simulink model "Backhoe_Arm"  (R2020a)
settings: Solver=ode23t  StartTime=0.0  StopTime=60  RelTol=1e-3  EnableMultiTasking=on
PostLoadFcn:
  | warning off simscape:compiler:sli:init:SolverNotRecommended
  | 
  | warning off sm:sli:visualization:UnsupportedSimMode
  | warning off sm:sli:setup:compile:LocalSolverNotSupported
  | warning off sm:compiler:state:UnsatisfiedDesiredTarget
  | 
  | warning off xPCTarget:sampleTime:sampleTimeInvariance
  | warning off Simulink:blocks:MatchingFromNotFound
model workspace (MAT data in the model file):
  cylinderGray = [0.6 0.6 0.6]
  darkOrange = [0.8 0.5 0]
  glassBlue = [0.2 0.2 1]
  gray = [0.3 0.3 0.3]
  orange = [0.8 0.65 0]
  pistonGray = [0.4 0.4 0.4]
  rhoGlass = 2500
  rhoRubber = 1500
  rhoSteel = 7800
  tireBlack = [0.1 0.1 0.1]
  wheelGray = [0.6 0.6 0.6]
  yellow = [0.8 0.8 0]
undefined symbols (not defined in the file or in its folder): BH_Param, sigbuilder_block, X, Y, Z
libraries: sm_lib x98, fl_lib x31, Backhoe_Lib x28, nesl_utility x22, sh_lib x9, slrtlib x1
(part 3 of 4)

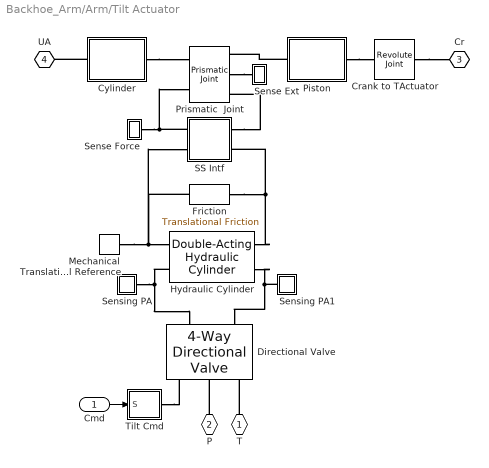
== system Backhoe_Arm/Arm/Tilt Actuator ==
  Cmd : Inport
  Crank to TActuator : sm_lib/Joints/Revolute Joint  JointMode=Normal  SenseConstraintForce=off  SenseConstraintForceX=off  SenseConstraintForceY=off  SenseConstraintForceZ=off  SenseConstraintTorque=off  SenseConstraintTorqueX=off  SenseConstraintTorqueY=off  SenseConstraintTorqueZ=off  SenseTotalForce=off  SenseTotalForceX=off  SenseTotalForceY=off  SenseTotalForceZ=off  SenseTotalTorque=off  SenseTotalTorqueX=off  SenseTotalTorqueY=off  SenseTotalTorqueZ=off  CompositeWrenchDir=FollowerOnBase  CompositeWrenchFrame=BaseFrame  EquilibriumPosition=0  EquilibriumPositionUnits=deg  SpringStiffness=0  SpringStiffnessUnits=N*m/deg  DampingCoefficient=0  DampingCoefficientUnits=N*m/(deg/s)  TorqueActuationMode=NoTorque  MotionActuationMode=ComputedMotion  SensePosition=off  SenseVelocity=off  SenseAcceleration=off  SenseTorqueForce=off  SenseLowerLimitTorqueForce=off  SenseUpperLimitTorqueForce=off  LowerLimitSpecify=off  LowerLimitBound=-90  LowerLimitBoundUnits=deg  LowerLimitStiffness=1e4  LowerLimitStiffnessUnits=N*m/deg  LowerLimitDamping=10  LowerLimitDampingUnits=N*m/(deg/s)  LowerLimitTransitionRegionWidth=0.1  LowerLimitTransitionRegionWidthUnits=deg  UpperLimitSpecify=off  UpperLimitBound=90  UpperLimitBoundUnits=deg  UpperLimitStiffness=1e4  UpperLimitStiffnessUnits=N*m/deg  UpperLimitDamping=10  UpperLimitDampingUnits=N*m/(deg/s)  UpperLimitTransitionRegionWidth=0.1  UpperLimitTransitionRegionWidthUnits=deg  PositionTargetSpecify=off  PositionTargetPriority=High  PositionTargetValue=0  PositionTargetValueUnits=deg  VelocityTargetSpecify=off  VelocityTargetPriority=High  VelocityTargetValue=0  VelocityTargetValueUnits=deg/s
  Cylinder : Subsystem
  Directional Valve : sh_lib/Valves/Directional Valves/4-Way Directional Valve  Tag=Factory Generic  area_spec=1  x_0_P_A=-1e-4 m  x_0_P_B=-1e-4 m  x_0_A_T=-1e-4 m  x_0_B_T=-1e-4 m  mdl_type_identical=1  mdl_type_different=1  opening_max=hydr_valve_max_opening m  area_max=hydr_valve_max_area mm^2  opening_max_P_A=0.005 m  area_max_P_A=0.5e-4 m^2  opening_max_P_B=0.005 m  area_max_P_B=0.5e-4 m^2  opening_max_A_T=0.005 m  area_max_A_T=0.5e-4 m^2  opening_max_B_T=0.005 m  area_max_B_T=0.5e-4 m^2  opening_area_tab="[  -0.002 0 0.005 0.015 ] m"  area_tab="[  1e-12 4e-12 1e-05 1.02e-05 ] m^2"  opening_flow_rate_tab="[  -0.002 0 0.005 0.015 ] m"  pressure_tab="[  -5e+06 -2e+06 2e+06 5e+06 ] Pa"  flow_rate_tab="[  -1e-12 -6e-14 6e+12 1e+11 ; -8e-08 -4e-08 4e+06 8e+06 ; -0.0025 -0.00103 0.001 0.0024 ; -0.00258 -0.001032 0.00106 0.00247 ; ] m^3/s"  opening_area_tab_P_A=[-0.002, 0.0, 0.002, 0.005, 0.015] m  area_tab_P_A=[1.0e-9, 2.0352e-7, 4.0736e-5, 0.00011438, 0.00034356] m^2  opening_flow_rate_tab_P_A=[-0.002, 0.0, 0.002, 0.005, 0.015] m  pressure_tab_P_A=[-10000000.0, -5000000.0, -2000000.0, 2000000.0, 5000000.0, 10000000.0] Pa  flow_rate_tab_P_A=[-1.0e-7, -7.0711e-8, -4.4721e-8, 4.4721e-8, 7.0711e-8, 1.0e-7; -2.0352e-5, -1.4391e-5, -9.1017e-6, 9.1017e-6, 1.4391e-5, 2.0352e-5; -0.0040736, -0.0028805, -0.0018218, 0.0018218, 0.0028805, 0.0040736; -0.011438, -0.0080879, -0.0051152, 0.0051152, 0.0080879, 0.011438; -0.034356, -0.024293, -0.015364, 0.015364, 0.024293, 0.034356] m^3/s  opening_area_tab_P_B=[-0.002, 0.0, 0.002, 0.005, 0.015] m  area_tab_P_B=[1.0e-9, 2.0352e-7, 4.0736e-5, 0.00011438, 0.00034356] m^2  opening_flow_rate_tab_P_B=[-0.002, 0.0, 0.002, 0.005, 0.015] m  pressure_tab_P_B=[-10000000.0, -5000000.0, -2000000.0, 2000000.0, 5000000.0, 10000000.0] Pa  flow_rate_tab_P_B=[-1.0e-7, -7.0711e-8, -4.4721e-8, 4.4721e-8, 7.0711e-8, 1.0e-7; -2.0352e-5, -1.4391e-5, -9.1017e-6, 9.1017e-6, 1.4391e-5, 2.0352e-5; -0.0040736, -0.0028805, -0.0018218, 0.0018218, 0.0028805, 0.0040736; -0.011438, -0.0080879, -0.0051152, 0.0051152, 0.0080879, 0.011438; -0.034356, -0.024293, -0.015364, 0.015364, 0.024293, 0.034356] m^3/s  opening_area_tab_A_T=[-0.002, 0.0, 0.002, 0.005, 0.015] m  area_tab_A_T=[1.0e-9, 2.0352e-7, 4.0736e-5, 0.00011438, 0.00034356] m^2  opening_flow_rate_tab_A_T=[-0.002, 0.0, 0.002, 0.005, 0.015] m  pressure_tab_A_T=[-10000000.0, -5000000.0, -2000000.0, 2000000.0, 5000000.0, 10000000.0] Pa  flow_rate_tab_A_T=[-1.0e-7, -7.0711e-8, -4.4721e-8, 4.4721e-8, 7.0711e-8, 1.0e-7; -2.0352e-5, -1.4391e-5, -9.1017e-6, 9.1017e-6, 1.4391e-5, 2.0352e-5; -0.0040736, -0.0028805, -0.0018218, 0.0018218, 0.0028805, 0.0040736; -0.011438, -0.0080879, -0.0051152, 0.0051152, 0.0080879, 0.011438; -0.034356, -0.024293, -0.015364, 0.015364, 0.024293, 0.034356] m^3/s  opening_area_tab_B_T=[-0.002, 0.0, 0.002, 0.005, 0.015] m  area_tab_B_T=[1.0e-9, 2.0352e-7, 4.0736e-5, 0.00011438, 0.00034356] m^2  opening_flow_rate_tab_B_T=[-0.002, 0.0, 0.002, 0.005, 0.015] m  pressure_tab_B_T=[-10000000.0, -5000000.0, -2000000.0, 2000000.0, 5000000.0, 10000000.0] Pa  flow_rate_tab_B_T=[-1.0e-7, -7.0711e-8, -4.4721e-8, 4.4721e-8, 7.0711e-8, 1.0e-7; -2.0352e-5, -1.4391e-5, -9.1017e-6, 9.1017e-6, 1.4391e-5, 2.0352e-5; -0.0040736, -0.0028805, -0.0018218, 0.0018218, 0.0028805, 0.0040736; -0.011438, -0.0080879, -0.0051152, 0.0051152, 0.0080879, 0.011438; -0.034356, -0.024293, -0.015364, 0.015364, 0.024293, 0.034356] m^3/s  interp_method_identical=1  interp_method_different=1  extrap_method_identical=1  extrap_method_different=1  A_leak=1e-12 m^2  C_d=0.7  lam_spec=2  B_lam=0.999  Re_cr=12
      settings: SourceProductBaseCode=SH  InternalSimscapePortConfiguration="{\"Bottom\":[],\"Left\":[{\"id\":\"A\",\"label\":\"A\",\"type\":\"foundation.hydraulic.hydraulic\"},{\"id\":\"B\",\"label\":\"B\",\"type\":\"foundation.hydraulic.hydraulic\"}],\"Right\":[{\"id\":\"S\",\"label\":\"S\",\"type\":\"input\"},{\"id\":\"P\",\"label\":\"P\",\"type\":\"foundation.hydraulic.hydraulic\"},{\"id\":\"T\",\"label\":\"T\",\"type\":\"foundation.hydraulic.hydraulic\"}],\"Top\":[]}"
  Friction : fl_lib/Mechanical/Translational Elements/Translational Friction  brkwy_frc=friction_breakaway N  brkwy_vel=0.060623 m/s  Col_frc=friction_coulomb N  visc_coef=friction_viscous N/(m/s)  v_specify=off  v_priority=High  v=0 m/s  v_nominal_specify=off  v_nominal_unit=m/s  v_nominal_value=1  f_specify=off  f_priority=High  f=0 N  f_nominal_specify=off  f_nominal_unit=N  f_nominal_value=1
      settings: SourceProductBaseCode=SS  InternalSimscapePortConfiguration="{\"Bottom\":[],\"Left\":[{\"id\":\"R\",\"label\":\"R\",\"type\":\"foundation.mechanical.translational.translational\"}],\"Right\":[{\"id\":\"C\",\"label\":\"C\",\"type\":\"foundation.mechanical.translational.translational\"}],\"Top\":[]}"
  Hydraulic Cylinder : sh_lib/Hydraulic Cylinders/Double-Acting Hydraulic Cylinder  Tag=Factory Generic  area_A=hydr_area m^2  area_B=hydr_area m^2  stroke=hydr_stroke m  init_pos=hydr_x0 m  dead_vol_A=hydr_deadvol m^3  dead_vol_B=hydr_deadvol m^3  init_pressure_A=hydr_PA0 Pa  init_pressure_B=hydr_PB0 Pa  k_sh=1.4  stiff=1e+06 N/m  D=150 N/(m/s)  hardstop_model=3  transition=0.1 mm  or=2
      settings: SourceProductBaseCode=SH  InternalSimscapePortConfiguration="{\"Bottom\":[],\"Left\":[{\"id\":\"C\",\"label\":\"C\",\"type\":\"foundation.mechanical.translational.translational\"},{\"id\":\"A\",\"label\":\"A\",\"type\":\"foundation.hydraulic.hydraulic\"}],\"Right\":[{\"id\":\"R\",\"label\":\"R\",\"type\":\"foundation.mechanical.translational.translational\"},{\"id\":\"B\",\"label\":\"B\",\"type\":\"foundation.hydraulic.hydraulic\"}],\"Top\":[]}"
  Mechanical Translational Reference : fl_lib/Mechanical/Translational Elements/Mechanical Translational Reference  Tag=Factory Generic
  Piston : Subsystem
  Prismatic  Joint : sm_lib/Joints/Prismatic Joint  JointMode=Normal  SenseConstraintForce=off  SenseConstraintForceX=off  SenseConstraintForceY=off  SenseConstraintForceZ=off  SenseConstraintTorque=off  SenseConstraintTorqueX=off  SenseConstraintTorqueY=off  SenseConstraintTorqueZ=off  SenseTotalForce=off  SenseTotalForceX=off  SenseTotalForceY=off  SenseTotalForceZ=off  SenseTotalTorque=off  SenseTotalTorqueX=off  SenseTotalTorqueY=off  SenseTotalTorqueZ=off  CompositeWrenchDir=FollowerOnBase  CompositeWrenchFrame=BaseFrame  EquilibriumPosition=0  EquilibriumPositionUnits=m  SpringStiffness=0  SpringStiffnessUnits=N/m  DampingCoefficient=0  DampingCoefficientUnits=N/(m/s)  TorqueActuationMode=InputTorque  MotionActuationMode=ComputedMotion  SensePosition=on  SenseVelocity=on  SenseAcceleration=off  SenseTorqueForce=off  SenseLowerLimitTorqueForce=off  SenseUpperLimitTorqueForce=off  LowerLimitSpecify=off  LowerLimitBound=-1  LowerLimitBoundUnits=m  LowerLimitStiffness=1e6  LowerLimitStiffnessUnits=N/m  LowerLimitDamping=1e3  LowerLimitDampingUnits=N/(m/s)  LowerLimitTransitionRegionWidth=1e-4  LowerLimitTransitionRegionWidthUnits=m  UpperLimitSpecify=off  UpperLimitBound=1  UpperLimitBoundUnits=m  UpperLimitStiffness=1e6  UpperLimitStiffnessUnits=N/m  UpperLimitDamping=1e3  UpperLimitDampingUnits=N/(m/s)  UpperLimitTransitionRegionWidth=1e-4  UpperLimitTransitionRegionWidthUnits=m  PositionTargetSpecify=off  PositionTargetPriority=Low  PositionTargetValue=0  PositionTargetValueUnits=m  VelocityTargetSpecify=off  VelocityTargetPriority=High  VelocityTargetValue=0  VelocityTargetValueUnits=m/s
  SS Intf : Subsystem
  Sense Ext : Subsystem
      mask Display: disp('S')
  Sense Force : Subsystem
      mask Display: disp('S')
  Sensing PA : Subsystem
      mask Display: disp('S')
  Sensing PA1 : Subsystem
      mask Display: disp('S')
  Tilt Cmd : Subsystem
  T : PMIOPort  Side=Left
  P : PMIOPort  Port=2  Side=Left
  Cr : PMIOPort  Port=3  Side=Right
  UA : PMIOPort  Port=4  Side=Right
  wires:
  Cmd/1 -> Tilt Cmd/1(S)
  connections:
  Crank to TActuator/RConn1 -- Cr/RConn1
  SS Intf/RConn1 -- Sense Force/RConn1 -- Prismatic  Joint/LConn2
  SS Intf/LConn1 -- Prismatic  Joint/RConn3
  Piston/LConn1 -- Prismatic  Joint/RConn1
  Cylinder/LConn1 -- Prismatic  Joint/LConn1
  Hydraulic Cylinder/RConn1 -- Friction/LConn1 -- SS Intf/LConn2
  Sensing PA/LConn1 -- Hydraulic Cylinder/LConn2 -- Directional Valve/LConn1
  Mechanical Translational Reference/LConn1 -- Friction/RConn1 -- SS Intf/RConn2 -- Hydraulic Cylinder/LConn1
  Hydraulic Cylinder/RConn2 -- Sensing PA1/LConn1 -- Directional Valve/LConn2
  Cylinder/RConn1 -- UA/RConn1
  P/RConn1 -- Directional Valve/RConn2
  T/RConn1 -- Directional Valve/RConn3
  Tilt Cmd/RConn1 -- Directional Valve/RConn1
  Prismatic  Joint/RConn2 -- Sense Ext/LConn1
  Piston/RConn1 -- Crank to TActuator/LConn1

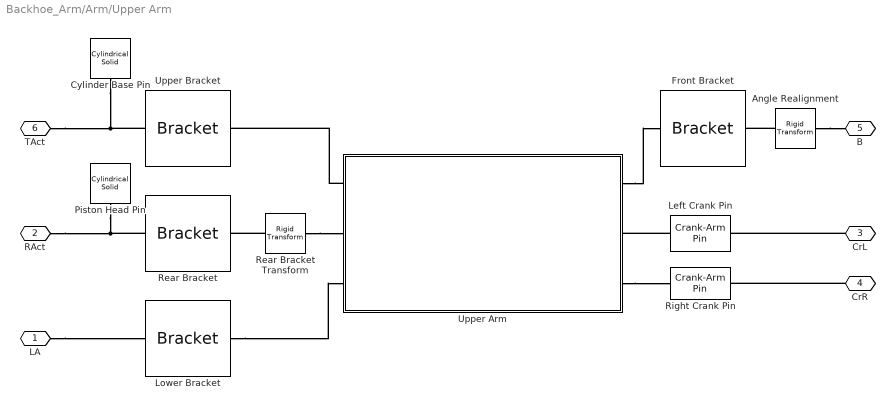
== system Backhoe_Arm/Arm/Upper Arm ==
  Angle Realignment : sm_lib/Frames and Transforms/Rigid Transform  TranslationMethod=None  TranslationStandardOffset=0  TranslationLengthUnit=m  TranslationStandardAxis=+Z  TranslationCartesianOffset=[0 0 0]  TranslationROffset=0  TranslationROffsetUnits=m  TranslationZOffset=0  TranslationZOffsetUnits=m  TranslationThetaOffset=0  TranslationThetaOffsetUnits=deg  RotationMethod=AlignedAxes  RotationAngleUnits=deg  RotationStandardAxis=-Z  RotationAngle=90  RotationArbitraryAxis=[0 0 1]  FollAlignAxisA=+X  BaseAlignAxisA=-Y  FollAlignAxisB=+Z  BaseAlignAxisB=+Z  RotationSequenceAxes=FollowerAxes  RotationSequence=XYX  RotationSequenceAngles=[0 0 0]  RotationSequenceAnglesUnits=deg  RotationMatrix=[1 0 0; 0 1 0; 0 0 1]
  Cylinder Base Pin : sm_lib/Body Elements/Cylindrical Solid  GraphicAmbientColor=[0.15 0.15 0.15 1.0]  BasedOnType=Density  CenterOfMass=[0 0 0]  CenterOfMassUnits=m  GraphicDiffuseColor=gray  CylinderLength=0.8  CylinderLengthUnits=m  CylinderRadius=0.075  CylinderRadiusUnits=m  Density=rhoSteel  DensityUnits=kg/(m^3)  DoExposeReferenceFrame=on  GraphicEmissiveColor=[0.0 0.0 0.0 1.0]  ExportEntireGeometry=off  SerializedFrames=<Frames/>  MarkerShape=Sphere  MarkerSize=10  GraphicType=FromGeometry  InertiaType=CalculateFromGeometry  Mass=1  MassUnits=kg  MomentsOfInertia=[1 1 1]  MomentsOfInertiaUnits=kg*m^2  GraphicOpacity=1.0  ProductsOfInertia=[0 0 0]  ProductsOfInertiaUnits=kg*m^2  GraphicShininess=75  GraphicSpecularColor=[0.5 0.5 0.5 1.0]  GraphicVisPropType=SimpleVisualProperties
  Front Bracket : Backhoe_Lib/Bracket  Hbracket=0.65  Wbracket=0.5  Tbracket=0.15  Dbracket=0.625  Hhole=0.4  Rhole=0.075  circlePoints=25  bracketColor=orange  rho=rhoSteel
  Left Crank Pin : Backhoe_Lib/Crank-Arm Pin  R=0.075  L=0.25  T=0.2  color=gray  rho=rhoSteel
  Lower Bracket : Backhoe_Lib/Bracket  Hbracket=0.75  Wbracket=0.75  Tbracket=0.15  Dbracket=0.75  Hhole=0.5  Rhole=0.075  circlePoints=25  bracketColor=orange  rho=rhoSteel
  Piston Head Pin : sm_lib/Body Elements/Cylindrical Solid  GraphicAmbientColor=[0.15 0.15 0.15 1.0]  BasedOnType=Density  CenterOfMass=[0 0 0]  CenterOfMassUnits=m  GraphicDiffuseColor=gray  CylinderLength=0.8  CylinderLengthUnits=m  CylinderRadius=0.075  CylinderRadiusUnits=m  Density=rhoSteel  DensityUnits=kg/(m^3)  DoExposeReferenceFrame=on  GraphicEmissiveColor=[0.0 0.0 0.0 1.0]  ExportEntireGeometry=off  SerializedFrames=<Frames/>  MarkerShape=Sphere  MarkerSize=10  GraphicType=FromGeometry  InertiaType=CalculateFromGeometry  Mass=1  MassUnits=kg  MomentsOfInertia=[1 1 1]  MomentsOfInertiaUnits=kg*m^2  GraphicOpacity=1.0  ProductsOfInertia=[0 0 0]  ProductsOfInertiaUnits=kg*m^2  GraphicShininess=75  GraphicSpecularColor=[0.5 0.5 0.5 1.0]  GraphicVisPropType=SimpleVisualProperties
  Rear Bracket : Backhoe_Lib/Bracket  Hbracket=0.75  Wbracket=0.75  Tbracket=0.15  Dbracket=0.75  Hhole=0.5  Rhole=0.075  circlePoints=25  bracketColor=orange  rho=rhoSteel
  Rear Bracket Transform : sm_lib/Frames and Transforms/Rigid Transform  TranslationMethod=None  TranslationStandardOffset=0.5  TranslationLengthUnit=m  TranslationStandardAxis=+Z  TranslationCartesianOffset=[ 0 0 0]  TranslationROffset=0  TranslationROffsetUnits=m  TranslationZOffset=0  TranslationZOffsetUnits=m  TranslationThetaOffset=0  TranslationThetaOffsetUnits=deg  RotationMethod=AlignedAxes  RotationAngleUnits=deg  RotationStandardAxis=+X  RotationAngle=90  RotationArbitraryAxis=[0 0 1]  FollAlignAxisA=+Z  BaseAlignAxisA=+Z  FollAlignAxisB=+Y  BaseAlignAxisB=-Y  RotationSequenceAxes=FollowerAxes  RotationSequence=XYX  RotationSequenceAngles=[0 0 0]  RotationSequenceAnglesUnits=deg  RotationMatrix=[1 0 0; 0 1 0; 0 0 1]
  Right Crank Pin : Backhoe_Lib/Crank-Arm Pin  R=0.075  L=0.25  T=0.2  color=gray  rho=rhoSteel
  Upper Arm : Subsystem  mask(Upper Arm){Lbar=6, Wbar=0.8, Tbar=0.85, L1=1.5, L2=1.5, L3=2.5, barFillet=0.1, numPoints=15, Tcrank=0.2, armColor=yellow, rho=rhoSteel}
      mask prompts: Lbar "Lbar [m]"; Wbar "Wbar [m]"; Tbar "Tbar [m]"; L1 "L1 [m]"; L2 "L2 [m]"; L3 "L3 [m]"; barFillet "Bar Fillet Radius [m]"; numPoints "Fillet Point Resolution"; Tcrank "Crank Arm Thickness [m]"; armColor "Arm Color"; rho "Density [kg/m^3]"
      mask help:
      | Consists of the backhoe upper arm and four attachment brackets -- front, rear, upper and lower.
      |
      | Attachment points are:
      | B: Bucket attachment.
      | CL: Crank arm attachment (Left).
      | CR: Crank arm attachment (Right).
      | BC: Bucket hydraulic actuator (Cylinder base).
      | LA: Lower Arm attachment.
      | UH: Upper arm hydraulic actuator (piston Head).
      | All attachment points are configured for Revolute joints.
      |
      | The lengths L1, L2 and L3 correspond to lengths measured from the center of the bar, as follows:
      | L1: Upper Bracket
      | L2: Lower Bracket
      | L3: Crank Attachment Points
      | The front and rear brackets are automatically placed at the center of the end faces of the upper arm bar.
      |
      | Click on Help to view a schematic of the upper arm, its configurable dimension parameters and attachment points (in red).
      mask init: same as Backhoe_Arm/Arm/Lower Arm /Lower Arm
      mask Help: web('Backhoe_Upperarm.html');
      mask DialogControl ParameterTabVar0 Prompt: General
      mask DialogControl ParameterTabVar01 Prompt: Material Properties
      mask Display:
      | image('Backhoe_Upperbar_IMAGE.png');
      | port_label('lconn',1,'CB');
      | port_label('lconn',2,'PH');
      | port_label('lconn',3,'LA');
      | port_label('rconn',1,'B');
      | port_label('rconn',2,'CL');
      | port_label('rconn',3,'CR');
  Upper Bracket : Backhoe_Lib/Bracket  Hbracket=0.75  Wbracket=0.75  Tbracket=0.15  Dbracket=0.75  Hhole=0.5  Rhole=0.075  circlePoints=25  bracketColor=orange  rho=rhoSteel
  LA : PMIOPort  Side=Left
  RAct : PMIOPort  Port=2  Side=Left
  CrL : PMIOPort  Port=3  Side=Right
  CrR : PMIOPort  Port=4  Side=Right
  B : PMIOPort  Port=5  Side=Right
  TAct : PMIOPort  Port=6  Side=Right
  connections:
  Cylinder Base Pin/RConn1 -- Upper Bracket/RConn1 -- TAct/RConn1
  Piston Head Pin/RConn1 -- RAct/RConn1 -- Rear Bracket/RConn1
  Angle Realignment/LConn1 -- Front Bracket/RConn1
  LA/RConn1 -- Lower Bracket/RConn1
  CrL/RConn1 -- Left Crank Pin/LConn1
  CrR/RConn1 -- Right Crank Pin/LConn1
  Rear Bracket Transform/RConn1 -- Rear Bracket/LConn1
  Upper Arm/LConn1 -- Upper Bracket/LConn1
  Upper Arm/RConn1 -- Front Bracket/LConn1
  Upper Arm/RConn3 -- Right Crank Pin/RConn1
  Lower Bracket/LConn1 -- Upper Arm/LConn3
  Rear Bracket Transform/LConn1 -- Upper Arm/LConn2
  Left Crank Pin/RConn1 -- Upper Arm/RConn2
  Angle Realignment/RConn1 -- B/RConn1

== system Backhoe_Arm/Arm/Bucket Assembly/Bucket ==
  Arm Revolute Rotation : sm_lib/Frames and Transforms/Rigid Transform  TranslationMethod=None  TranslationStandardOffset=0  TranslationLengthUnit=m  TranslationStandardAxis=+X  TranslationCartesianOffset=[0 0 0]  TranslationROffset=0  TranslationROffsetUnits=m  TranslationZOffset=0  TranslationZOffsetUnits=m  TranslationThetaOffset=0  TranslationThetaOffsetUnits=deg  RotationMethod=AlignedAxes  RotationAngleUnits=deg  RotationStandardAxis=-Y  RotationAngle=180  RotationArbitraryAxis=[0 0 1]  FollAlignAxisA=+Y  BaseAlignAxisA=+Y  FollAlignAxisB=+X  BaseAlignAxisB=-X  RotationSequenceAxes=FollowerAxes  RotationSequence=XYX  RotationSequenceAngles=[0 0 0]  RotationSequenceAnglesUnits=deg  RotationMatrix=[1 0 0; 0 1 0; 0 0 1]
  Attachment Frame : Subsystem
      mask Display:
      | image('Backhoe_Attach_IMAGE.png');
      | port_label('lconn',1,'B');
      | port_label('rconn',1,'CA');
      | port_label('rconn',2,'UA');
  Bucket : Subsystem
      mask Display:
      | image('Backhoe_Bucketcase_IMAGE.png');
      | port_label('rconn',1,'AF');
  Crank Revolute Rotation : sm_lib/Frames and Transforms/Rigid Transform  TranslationMethod=None  TranslationStandardOffset=0  TranslationLengthUnit=m  TranslationStandardAxis=+X  TranslationCartesianOffset=[0 0 0]  TranslationROffset=0  TranslationROffsetUnits=m  TranslationZOffset=0  TranslationZOffsetUnits=m  TranslationThetaOffset=0  TranslationThetaOffsetUnits=deg  RotationMethod=AlignedAxes  RotationAngleUnits=deg  RotationStandardAxis=-Y  RotationAngle=180  RotationArbitraryAxis=[0 0 1]  FollAlignAxisA=+Y  BaseAlignAxisA=+Y  FollAlignAxisB=+X  BaseAlignAxisB=-X  RotationSequenceAxes=FollowerAxes  RotationSequence=XYX  RotationSequenceAngles=[0 0 0]  RotationSequenceAnglesUnits=deg  RotationMatrix=[1 0 0; 0 1 0; 0 0 1]
  Crank Arm : PMIOPort  Side=Right
  Upper Arm : PMIOPort  Port=2  Side=Right
  connections:
  Bucket/RConn1 -- Attachment Frame/LConn1
  Crank Revolute Rotation/LConn1 -- Attachment Frame/RConn1
  Arm Revolute Rotation/LConn1 -- Attachment Frame/RConn2
  Upper Arm/RConn1 -- Arm Revolute Rotation/RConn1
  Crank Arm/RConn1 -- Crank Revolute Rotation/RConn1

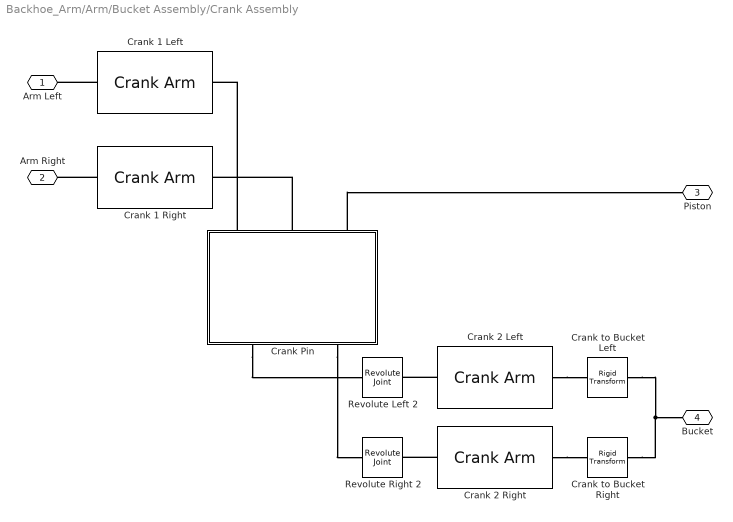
== system Backhoe_Arm/Arm/Bucket Assembly/Crank Assembly ==
  Crank 1 Left : Backhoe_Lib/Crank Arm  L=LC1  W=WC1  T=TC1  D=DH1  R=Rpin  Nc=25  color=color1  rho=rho1
  Crank 1 Right : Backhoe_Lib/Crank Arm  L=LC1  W=WC1  T=TC1  D=DH1  R=Rpin  Nc=25  color=color1  rho=rho1
  Crank 2 Left : Backhoe_Lib/Crank Arm  L=LC2  W=WC2  T=TC2  D=DH2  R=Rpin  Nc=25  color=color2  rho=rho2
  Crank 2 Right : Backhoe_Lib/Crank Arm  L=LC2  W=WC2  T=TC2  D=DH2  R=Rpin  Nc=25  color=color2  rho=rho2
  Crank Pin : Subsystem
      mask Display:
      | image(repmat(imread('Backhoe_Crankpin_IMAGE.png'),[1 1 3]));
      | port_label('lconn',1,'C1L');
      | port_label('lconn',2,'C2L');
      | port_label('lconn',3,'PA');
      | port_label('rconn',1,'C2L');
      | port_label('rconn',2,'C2R');
  Crank to Bucket Right : sm_lib/Frames and Transforms/Rigid Transform  TranslationMethod=StandardAxis  TranslationStandardOffset=(DC2 - TC2)/2  TranslationLengthUnit=m  TranslationStandardAxis=+Z  TranslationCartesianOffset=[0 0 0]  TranslationROffset=0  TranslationROffsetUnits=m  TranslationZOffset=0  TranslationZOffsetUnits=m  TranslationThetaOffset=0  TranslationThetaOffsetUnits=deg  RotationMethod=None  RotationAngleUnits=deg  RotationStandardAxis=+Z  RotationAngle=0  RotationArbitraryAxis=[0 0 1]  FollAlignAxisA=+X  BaseAlignAxisA=+Y  FollAlignAxisB=+Y  BaseAlignAxisB=+Z  RotationSequenceAxes=FollowerAxes  RotationSequence=XYX  RotationSequenceAngles=[0 0 0]  RotationSequenceAnglesUnits=deg  RotationMatrix=[1 0 0; 0 1 0; 0 0 1]
  Crank to Bucket Left : sm_lib/Frames and Transforms/Rigid Transform  TranslationMethod=StandardAxis  TranslationStandardOffset=(DC2 - TC2)/2  TranslationLengthUnit=m  TranslationStandardAxis=-Z  TranslationCartesianOffset=[0 0 0]  TranslationROffset=0  TranslationROffsetUnits=m  TranslationZOffset=0  TranslationZOffsetUnits=m  TranslationThetaOffset=0  TranslationThetaOffsetUnits=deg  RotationMethod=None  RotationAngleUnits=deg  RotationStandardAxis=+Z  RotationAngle=0  RotationArbitraryAxis=[0 0 1]  FollAlignAxisA=+X  BaseAlignAxisA=+Y  FollAlignAxisB=+Y  BaseAlignAxisB=+Z  RotationSequenceAxes=FollowerAxes  RotationSequence=XYX  RotationSequenceAngles=[0 0 0]  RotationSequenceAnglesUnits=deg  RotationMatrix=[1 0 0; 0 1 0; 0 0 1]
  Revolute Left 2 : sm_lib/Joints/Revolute Joint  JointMode=Normal  SenseConstraintForce=off  SenseConstraintForceX=off  SenseConstraintForceY=off  SenseConstraintForceZ=off  SenseConstraintTorque=off  SenseConstraintTorqueX=off  SenseConstraintTorqueY=off  SenseConstraintTorqueZ=off  SenseTotalForce=off  SenseTotalForceX=off  SenseTotalForceY=off  SenseTotalForceZ=off  SenseTotalTorque=off  SenseTotalTorqueX=off  SenseTotalTorqueY=off  SenseTotalTorqueZ=off  CompositeWrenchDir=FollowerOnBase  CompositeWrenchFrame=BaseFrame  EquilibriumPosition=0  EquilibriumPositionUnits=deg  SpringStiffness=0  SpringStiffnessUnits=N*m/deg  DampingCoefficient=0  DampingCoefficientUnits=N*m/(deg/s)  TorqueActuationMode=NoTorque  MotionActuationMode=ComputedMotion  SensePosition=off  SenseVelocity=off  SenseAcceleration=off  SenseTorqueForce=off  SenseLowerLimitTorqueForce=off  SenseUpperLimitTorqueForce=off  LowerLimitSpecify=off  LowerLimitBound=-90  LowerLimitBoundUnits=deg  LowerLimitStiffness=1e4  LowerLimitStiffnessUnits=N*m/deg  LowerLimitDamping=10  LowerLimitDampingUnits=N*m/(deg/s)  LowerLimitTransitionRegionWidth=0.1  LowerLimitTransitionRegionWidthUnits=deg  UpperLimitSpecify=off  UpperLimitBound=90  UpperLimitBoundUnits=deg  UpperLimitStiffness=1e4  UpperLimitStiffnessUnits=N*m/deg  UpperLimitDamping=10  UpperLimitDampingUnits=N*m/(deg/s)  UpperLimitTransitionRegionWidth=0.1  UpperLimitTransitionRegionWidthUnits=deg  PositionTargetSpecify=off  PositionTargetPriority=Low  PositionTargetValue=-45  PositionTargetValueUnits=deg  VelocityTargetSpecify=off  VelocityTargetPriority=High  VelocityTargetValue=0  VelocityTargetValueUnits=deg/s
  Revolute Right 2 : sm_lib/Joints/Revolute Joint  JointMode=Normal  SenseConstraintForce=off  SenseConstraintForceX=off  SenseConstraintForceY=off  SenseConstraintForceZ=off  SenseConstraintTorque=off  SenseConstraintTorqueX=off  SenseConstraintTorqueY=off  SenseConstraintTorqueZ=off  SenseTotalForce=off  SenseTotalForceX=off  SenseTotalForceY=off  SenseTotalForceZ=off  SenseTotalTorque=off  SenseTotalTorqueX=off  SenseTotalTorqueY=off  SenseTotalTorqueZ=off  CompositeWrenchDir=FollowerOnBase  CompositeWrenchFrame=BaseFrame  EquilibriumPosition=0  EquilibriumPositionUnits=deg  SpringStiffness=0  SpringStiffnessUnits=N*m/deg  DampingCoefficient=0  DampingCoefficientUnits=N*m/(deg/s)  TorqueActuationMode=NoTorque  MotionActuationMode=ComputedMotion  SensePosition=off  SenseVelocity=off  SenseAcceleration=off  SenseTorqueForce=off  SenseLowerLimitTorqueForce=off  SenseUpperLimitTorqueForce=off  LowerLimitSpecify=off  LowerLimitBound=-90  LowerLimitBoundUnits=deg  LowerLimitStiffness=1e4  LowerLimitStiffnessUnits=N*m/deg  LowerLimitDamping=10  LowerLimitDampingUnits=N*m/(deg/s)  LowerLimitTransitionRegionWidth=0.1  LowerLimitTransitionRegionWidthUnits=deg  UpperLimitSpecify=off  UpperLimitBound=90  UpperLimitBoundUnits=deg  UpperLimitStiffness=1e4  UpperLimitStiffnessUnits=N*m/deg  UpperLimitDamping=10  UpperLimitDampingUnits=N*m/(deg/s)  UpperLimitTransitionRegionWidth=0.1  UpperLimitTransitionRegionWidthUnits=deg  PositionTargetSpecify=off  PositionTargetPriority=High  PositionTargetValue=0  PositionTargetValueUnits=deg  VelocityTargetSpecify=off  VelocityTargetPriority=High  VelocityTargetValue=0  VelocityTargetValueUnits=deg/s
  Arm Left : PMIOPort  Side=Left
  Arm Right : PMIOPort  Port=2  Side=Left
  Piston : PMIOPort  Port=3  Side=Right
  Bucket : PMIOPort  Port=4  Side=Right
  connections:
  Crank Pin/RConn1 -- Revolute Left 2/LConn1
  Crank Pin/RConn2 -- Revolute Right 2/LConn1
  Crank 2 Left/LConn1 -- Revolute Left 2/RConn1
  Crank to Bucket Right/RConn1 -- Crank to Bucket Left/RConn1 -- Bucket/RConn1
  Crank Pin/LConn3 -- Piston/RConn1
  Crank 1 Left/RConn1 -- Arm Left/RConn1
  Crank 1 Right/RConn1 -- Arm Right/RConn1
  Crank Pin/LConn1 -- Crank 1 Left/LConn1
  Crank Pin/LConn2 -- Crank 1 Right/LConn1
  Crank 2 Right/LConn1 -- Revolute Right 2/RConn1
  Crank 2 Right/RConn1 -- Crank to Bucket Right/LConn1
  Crank 2 Left/RConn1 -- Crank to Bucket Left/LConn1

== system Backhoe_Arm/Arm/Lift Actuator/Cylinder ==
  Base to Cylinder Transform : sm_lib/Frames and Transforms/Rigid Transform  TranslationMethod=StandardAxis  TranslationStandardOffset=(Lcyl/2)  TranslationLengthUnit=m  TranslationStandardAxis=-Z  TranslationCartesianOffset=[0 0 0]  TranslationROffset=0  TranslationROffsetUnits=m  TranslationZOffset=0  TranslationZOffsetUnits=m  TranslationThetaOffset=0  TranslationThetaOffsetUnits=deg  RotationMethod=AlignedAxes  RotationAngleUnits=deg  RotationStandardAxis=+X  RotationAngle=90  RotationArbitraryAxis=[0 0 1]  FollAlignAxisA=+X  BaseAlignAxisA=+X  FollAlignAxisB=+Z  BaseAlignAxisB=-Z  RotationSequenceAxes=FollowerAxes  RotationSequence=XYX  RotationSequenceAngles=[0 0 0]  RotationSequenceAnglesUnits=deg  RotationMatrix=[1 0 0; 0 1 0; 0 0 1]
  Cylinder : sm_lib/Body Elements/Extruded Solid  GraphicAmbientColor=[0.15 0.15 0.15 1.0]  BasedOnType=Density  CenterOfMass=[0 0 0]  CenterOfMassUnits=m  GraphicDiffuseColor=cylColor  ExportConvexHullGeometry=off  ExtrusionCrossSection=cylSection  ExtrusionCrossSectionUnits=m  Density=rhoCyl  DensityUnits=kg/(m^3)  DoExposeReferenceFrame=on  GraphicEmissiveColor=[0.0 0.0 0.0 1.0]  ExportEntireGeometry=off  ExtrusionLength=Lcyl  ExtrusionLengthUnits=m  ExtrusionType=General  SerializedFrames=<Frames/>  MarkerShape=Sphere  MarkerSize=10  GraphicType=FromGeometry  InertiaType=CalculateFromGeometry  Mass=1  MassUnits=kg  MomentsOfInertia=[1 1 1]  MomentsOfInertiaUnits=kg*m^2  PolygonNumSides=3  GraphicOpacity=1  PolygonOuterRadius=1  PolygonOuterRadiusUnits=m  ProductsOfInertia=[0 0 0]  ProductsOfInertiaUnits=kg*m^2  GraphicShininess=75  GraphicSpecularColor=[0.5 0.5 0.5 1.0]  GraphicVisPropType=SimpleVisualProperties
  Single Bracket : Backhoe_Lib/Single Bracket  Hbracket=Lbase  Wbracket=Wbase  Tbracket=Wbase  Hhole=Lbase-(Wbase/2)  Rhole=Rbp  Nc=25  bracketColor=connColor  rho=rhoConn
  F : PMIOPort  Side=Right
  B : PMIOPort  Port=2  Side=Left
  connections:
  Single Bracket/RConn1 -- F/RConn1
  Single Bracket/LConn1 -- Base to Cylinder Transform/RConn1
  Cylinder/RConn1 -- Base to Cylinder Transform/LConn1 -- B/RConn1

== system Backhoe_Arm/Arm/Lift Actuator/Lift ==
  S : Inport
  Lift Cmd : Selector  InputPortWidth=3  IndexOptions=Index vector (dialog)  Indices=3  OutputSizes=1
  Simulink-PS Converter : nesl_utility/Simulink-PS Converter  PhysicalDomain=network_engine_domain  SubClassName=ps_input  LeftPortType=input  RightPortType=output  PseudoPeriodic=off  Frequencies=[]  NoiseDistribution=none  NoiseParameters=[]  Unit=1  AffineConversion=off  FilteringAndDerivatives=zero  SimscapeFilterOrder=1  InputFilterTimeConstant=0.005  UdotUserProvided=0
  PS : PMIOPort  Side=Right
  wires:
  Lift Cmd/1 -> Simulink-PS Converter/1
  S/1 -> Lift Cmd/1
  connections:
  PS/RConn1 -- Simulink-PS Converter/RConn1

== system Backhoe_Arm/Arm/Lift Actuator/Piston ==
  Piston : sm_lib/Body Elements/Cylindrical Solid  GraphicAmbientColor=[0.15 0.15 0.15 1.0]  BasedOnType=Density  CenterOfMass=[0 0 0]  CenterOfMassUnits=m  GraphicDiffuseColor=pistColor  CylinderLength=Lpist  CylinderLengthUnits=m  CylinderRadius=Rpist  CylinderRadiusUnits=m  Density=rhoPist  DensityUnits=kg/(m^3)  DoExposeReferenceFrame=on  GraphicEmissiveColor=[0.0 0.0 0.0 1.0]  ExportEntireGeometry=off  SerializedFrames=<Frames/>  MarkerShape=Sphere  MarkerSize=10  GraphicType=FromGeometry  InertiaType=CalculateFromGeometry  Mass=1  MassUnits=kg  MomentsOfInertia=[1 1 1]  MomentsOfInertiaUnits=kg*m^2  GraphicOpacity=1.0  ProductsOfInertia=[0 0 0]  ProductsOfInertiaUnits=kg*m^2  GraphicShininess=75  GraphicSpecularColor=[0.5 0.5 0.5 1.0]  GraphicVisPropType=SimpleVisualProperties
  Piston to Head Transform : sm_lib/Frames and Transforms/Rigid Transform  TranslationMethod=StandardAxis  TranslationStandardOffset=Lpist/2  TranslationLengthUnit=m  TranslationStandardAxis=+Z  TranslationCartesianOffset=[0 0 0]  TranslationROffset=0  TranslationROffsetUnits=m  TranslationZOffset=0  TranslationZOffsetUnits=m  TranslationThetaOffset=0  TranslationThetaOffsetUnits=deg  RotationMethod=AlignedAxes  RotationAngleUnits=deg  RotationStandardAxis=-X  RotationAngle=90  RotationArbitraryAxis=[0 0 1]  FollAlignAxisA=+Y  BaseAlignAxisA=-Y  FollAlignAxisB=+Z  BaseAlignAxisB=+Z  RotationSequenceAxes=FollowerAxes  RotationSequence=XYX  RotationSequenceAngles=[0 0 0]  RotationSequenceAnglesUnits=deg  RotationMatrix=[1 0 0; 0 1 0; 0 0 1]
  Single Bracket : Backhoe_Lib/Single Bracket  Hbracket=Lbase  Wbracket=Wbase  Tbracket=Whead  Hhole=Lhead-(Whead/2)  Rhole=Rhp  Nc=25  bracketColor=connColor  rho=rhoConn
  B : PMIOPort  Side=Left
  F : PMIOPort  Port=2  Side=Right
  connections:
  Single Bracket/RConn1 -- F/RConn1
  Piston to Head Transform/RConn1 -- Single Bracket/LConn1
  B/RConn1 -- Piston to Head Transform/LConn1 -- Piston/RConn1

== system Backhoe_Arm/Arm/Lift Actuator/SS Intf ==
  Ideal Force Sensor : fl_lib/Mechanical/Mechanical Sensors/Ideal Force Sensor
  Ideal Translational Velocity Source : fl_lib/Mechanical/Mechanical Sources/Ideal Translational Velocity Source
  F : PMIOPort  Side=Right
  V : PMIOPort  Port=2  Side=Left
  R : PMIOPort  Port=3  Side=Left
  C : PMIOPort  Port=4  Side=Right
  connections:
  Ideal Force Sensor/RConn2 -- F/RConn1
  Ideal Force Sensor/LConn1 -- R/RConn1
  C/RConn1 -- Ideal Translational Velocity Source/RConn2
  V/RConn1 -- Ideal Translational Velocity Source/RConn1
  Ideal Force Sensor/RConn1 -- Ideal Translational Velocity Source/LConn1

== system Backhoe_Arm/Arm/Lift Actuator/Sense Ext ==
  PS-Simulink Converter : nesl_utility/PS-Simulink Converter  PhysicalDomain=network_engine_domain  SubClassName=ps_output  LeftPortType=input  RightPortType=output  PseudoPeriodic=off  Frequencies=[]  Unit=1  AffineConversion=off
  Conn1 : PMIOPort  Side=Left
  tag scope: Lift_Ext=global
  wires:
  PS-Simulink Converter/1 -> [Lift_Ext]
  connections:
  Conn1/RConn1 -- PS-Simulink Converter/LConn1

== system Backhoe_Arm/Arm/Lift Actuator/Sense Force ==
  PS-Simulink Converter : nesl_utility/PS-Simulink Converter  PhysicalDomain=network_engine_domain  SubClassName=ps_output  LeftPortType=input  RightPortType=output  PseudoPeriodic=off  Frequencies=[]  Unit=1  AffineConversion=off
  S : PMIOPort  Side=Right
  tag scope: Lift_Force=global
  wires:
  PS-Simulink Converter/1 -> [Lift_Force]
  connections:
  PS-Simulink Converter/LConn1 -- S/RConn1

== system Backhoe_Arm/Arm/Lift Actuator/Sensing PA ==
  Hydraulic Pressure Sensor : fl_lib/Hydraulic/Hydraulic Sensors/Hydraulic Pressure Sensor
  Hydraulic Reference : fl_lib/Hydraulic/Hydraulic Elements/Hydraulic Reference
  PS-Simulink Converter1 : nesl_utility/PS-Simulink Converter  PhysicalDomain=network_engine_domain  SubClassName=ps_output  LeftPortType=input  RightPortType=output  PseudoPeriodic=off  Frequencies=[]  Unit=Pa  AffineConversion=off
  A : PMIOPort  Side=Left
  tag scope: Lift_PA=global
  wires:
  PS-Simulink Converter1/1 -> [Lift_PA]
  connections:
  Hydraulic Pressure Sensor/LConn1 -- A/RConn1
  Hydraulic Reference/LConn1 -- Hydraulic Pressure Sensor/RConn1
  PS-Simulink Converter1/LConn1 -- Hydraulic Pressure Sensor/RConn2

== system Backhoe_Arm/Arm/Lift Actuator/Sensing PA1 ==
  Hydraulic Pressure Sensor : fl_lib/Hydraulic/Hydraulic Sensors/Hydraulic Pressure Sensor
  Hydraulic Reference1 : fl_lib/Hydraulic/Hydraulic Elements/Hydraulic Reference
  PS-Simulink Converter1 : nesl_utility/PS-Simulink Converter  PhysicalDomain=network_engine_domain  SubClassName=ps_output  LeftPortType=input  RightPortType=output  PseudoPeriodic=off  Frequencies=[]  Unit=Pa  AffineConversion=off
  A : PMIOPort  Side=Left
  tag scope: Lift_PB=global
  wires:
  PS-Simulink Converter1/1 -> [Lift_PB]
  connections:
  PS-Simulink Converter1/LConn1 -- Hydraulic Pressure Sensor/RConn2
  Hydraulic Reference1/LConn1 -- Hydraulic Pressure Sensor/RConn1
  Hydraulic Pressure Sensor/LConn1 -- A/RConn1

== system Backhoe_Arm/Arm/Lower Arm /Lower Arm ==
  Bar : sm_lib/Body Elements/Extruded Solid  GraphicAmbientColor=[0.15 0.15 0.15 1.0]  BasedOnType=Density  CenterOfMass=[0 0 0]  CenterOfMassUnits=m  GraphicDiffuseColor=armColor  ExportConvexHullGeometry=off  ExtrusionCrossSection=barSection  ExtrusionCrossSectionUnits=m  Density=rho  DensityUnits=kg/(m^3)  DoExposeReferenceFrame=on  GraphicEmissiveColor=[0.0 0.0 0.0 1.0]  ExportEntireGeometry=off  ExtrusionLength=Lbar  ExtrusionLengthUnits=m  ExtrusionType=General  SerializedFrames=<Frames/>  MarkerShape=Sphere  MarkerSize=10  GraphicType=FromGeometry  InertiaType=CalculateFromGeometry  Mass=1  MassUnits=kg  MomentsOfInertia=[1 1 1]  MomentsOfInertiaUnits=kg*m^2  PolygonNumSides=3  GraphicOpacity=1.0  PolygonOuterRadius=1  PolygonOuterRadiusUnits=m  ProductsOfInertia=[0 0 0]  ProductsOfInertiaUnits=kg*m^2  GraphicShininess=75  GraphicSpecularColor=[0.5 0.5 0.5 1.0]  GraphicVisPropType=SimpleVisualProperties
  Front Bracket Transform : sm_lib/Frames and Transforms/Rigid Transform  TranslationMethod=StandardAxis  TranslationStandardOffset=Lbar/2  TranslationLengthUnit=m  TranslationStandardAxis=+Z  TranslationCartesianOffset=[0 0 0]  TranslationROffset=0  TranslationROffsetUnits=m  TranslationZOffset=0  TranslationZOffsetUnits=m  TranslationThetaOffset=0  TranslationThetaOffsetUnits=deg  RotationMethod=None  RotationAngleUnits=deg  RotationStandardAxis=-Y  RotationAngle=90  RotationArbitraryAxis=[0 0 1]  FollAlignAxisA=+X  BaseAlignAxisA=+Y  FollAlignAxisB=+Y  BaseAlignAxisB=+Z  RotationSequenceAxes=FollowerAxes  RotationSequence=XYX  RotationSequenceAngles=[0 0 0]  RotationSequenceAnglesUnits=deg  RotationMatrix=[1 0 0; 0 1 0; 0 0 1]
  Rear Bracket Transform : sm_lib/Frames and Transforms/Rigid Transform  TranslationMethod=StandardAxis  TranslationStandardOffset=Lbar/2  TranslationLengthUnit=m  TranslationStandardAxis=-Z  TranslationCartesianOffset=[0 0 0]  TranslationROffset=0  TranslationROffsetUnits=m  TranslationZOffset=0  TranslationZOffsetUnits=m  TranslationThetaOffset=0  TranslationThetaOffsetUnits=deg  RotationMethod=AlignedAxes  RotationAngleUnits=deg  RotationStandardAxis=+Y  RotationAngle=180  RotationArbitraryAxis=[0 0 1]  FollAlignAxisA=+Y  BaseAlignAxisA=+Y  FollAlignAxisB=+X  BaseAlignAxisB=-X  RotationSequenceAxes=FollowerAxes  RotationSequence=XYX  RotationSequenceAngles=[0 0 0]  RotationSequenceAnglesUnits=deg  RotationMatrix=[1 0 0; 0 1 0; 0 0 1]
  Upper Bracket Transform : sm_lib/Frames and Transforms/Rigid Transform  TranslationMethod=Cartesian  TranslationStandardOffset=Lbar/2  TranslationLengthUnit=m  TranslationStandardAxis=-X  TranslationCartesianOffset=[Tbar/2 0 Lb]  TranslationROffset=0  TranslationROffsetUnits=m  TranslationZOffset=0  TranslationZOffsetUnits=m  TranslationThetaOffset=0  TranslationThetaOffsetUnits=deg  RotationMethod=AlignedAxes  RotationAngleUnits=deg  RotationStandardAxis=+Y  RotationAngle=90  RotationArbitraryAxis=[0 0 1]  FollAlignAxisA=+Y  BaseAlignAxisA=-Y  FollAlignAxisB=+Z  BaseAlignAxisB=+X  RotationSequenceAxes=FollowerAxes  RotationSequence=XYX  RotationSequenceAngles=[0 0 0]  RotationSequenceAnglesUnits=deg  RotationMatrix=[1 0 0; 0 1 0; 0 0 1]
  Rear Bracket : PMIOPort  Side=Right
  Upper Bracket : PMIOPort  Port=2  Side=Left
  Front Bracket : PMIOPort  Port=3  Side=Left
  connections:
  Upper Bracket/RConn1 -- Upper Bracket Transform/RConn1
  Rear Bracket Transform/RConn1 -- Rear Bracket/RConn1
  Front Bracket Transform/RConn1 -- Front Bracket/RConn1
  Upper Bracket Transform/LConn1 -- Bar/RConn1 -- Rear Bracket Transform/LConn1 -- Front Bracket Transform/LConn1

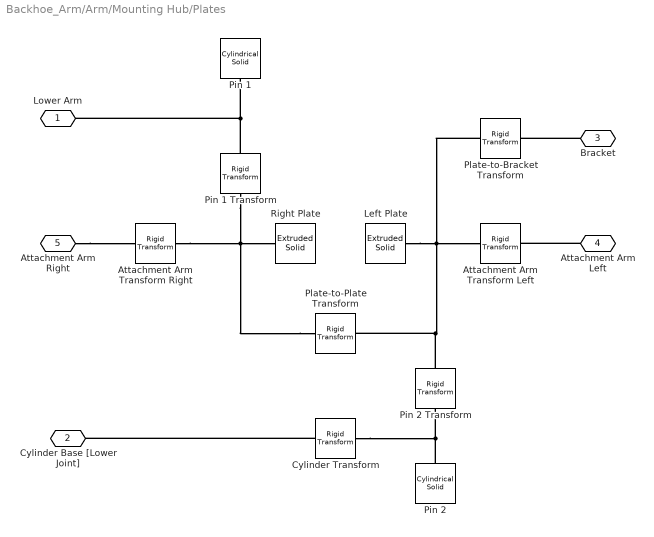
== system Backhoe_Arm/Arm/Mounting Hub/Plates ==
  Attachment Arm Transform Left : sm_lib/Frames and Transforms/Rigid Transform  TranslationMethod=Cartesian  TranslationStandardOffset=Dplates  TranslationLengthUnit=m  TranslationStandardAxis=-Z  TranslationCartesianOffset=[L3 H3 (Larm-Warm+Tplate)/2]  TranslationROffset=0  TranslationROffsetUnits=m  TranslationZOffset=0  TranslationZOffsetUnits=m  TranslationThetaOffset=0  TranslationThetaOffsetUnits=deg  RotationMethod=None  RotationAngleUnits=deg  RotationStandardAxis=+Y  RotationAngle=90  RotationArbitraryAxis=[0 0 1]  FollAlignAxisA=+X  BaseAlignAxisA=+Y  FollAlignAxisB=+Y  BaseAlignAxisB=+Z  RotationSequenceAxes=FollowerAxes  RotationSequence=XYX  RotationSequenceAngles=[0 0 0]  RotationSequenceAnglesUnits=deg  RotationMatrix=[1 0 0; 0 1 0; 0 0 1]
  Attachment Arm Transform Right : sm_lib/Frames and Transforms/Rigid Transform  TranslationMethod=Cartesian  TranslationStandardOffset=Dplates  TranslationLengthUnit=m  TranslationStandardAxis=-Z  TranslationCartesianOffset=[L3 H3 -(Larm-Warm+Tplate)/2]  TranslationROffset=0  TranslationROffsetUnits=m  TranslationZOffset=0  TranslationZOffsetUnits=m  TranslationThetaOffset=0  TranslationThetaOffsetUnits=deg  RotationMethod=None  RotationAngleUnits=deg  RotationStandardAxis=+Y  RotationAngle=90  RotationArbitraryAxis=[0 0 1]  FollAlignAxisA=+X  BaseAlignAxisA=+Y  FollAlignAxisB=+Y  BaseAlignAxisB=+Z  RotationSequenceAxes=FollowerAxes  RotationSequence=XYX  RotationSequenceAngles=[0 0 0]  RotationSequenceAnglesUnits=deg  RotationMatrix=[1 0 0; 0 1 0; 0 0 1]
  Cylinder Transform : sm_lib/Frames and Transforms/Rigid Transform  TranslationMethod=None  TranslationStandardOffset=0  TranslationLengthUnit=m  TranslationStandardAxis=+Z  TranslationCartesianOffset=[0 0 0]  TranslationROffset=0  TranslationROffsetUnits=m  TranslationZOffset=0  TranslationZOffsetUnits=m  TranslationThetaOffset=0  TranslationThetaOffsetUnits=deg  RotationMethod=AlignedAxes  RotationAngleUnits=deg  RotationStandardAxis=+Z  RotationAngle=0  RotationArbitraryAxis=[0 0 1]  FollAlignAxisA=+Z  BaseAlignAxisA=-Z  FollAlignAxisB=+X  BaseAlignAxisB=+X  RotationSequenceAxes=FollowerAxes  RotationSequence=XYX  RotationSequenceAngles=[0 0 0]  RotationSequenceAnglesUnits=deg  RotationMatrix=[1 0 0; 0 1 0; 0 0 1]
  Left Plate : sm_lib/Body Elements/Extruded Solid  GraphicAmbientColor=[0.15 0.15 0.15 1.0]  BasedOnType=Density  CenterOfMass=[0 0 0]  CenterOfMassUnits=m  GraphicDiffuseColor=hubColor  ExportConvexHullGeometry=off  ExtrusionCrossSection=plateSection  ExtrusionCrossSectionUnits=m  Density=rho  DensityUnits=kg/(m^3)  DoExposeReferenceFrame=on  GraphicEmissiveColor=[0.0 0.0 0.0 1.0]  ExportEntireGeometry=off  ExtrusionLength=Tplate  ExtrusionLengthUnits=m  ExtrusionType=General  SerializedFrames=<Frames/>  MarkerShape=Sphere  MarkerSize=10  GraphicType=FromGeometry  InertiaType=CalculateFromGeometry  Mass=1  MassUnits=kg  MomentsOfInertia=[1 1 1]  MomentsOfInertiaUnits=kg*m^2  PolygonNumSides=3  GraphicOpacity=1.0  PolygonOuterRadius=1  PolygonOuterRadiusUnits=m  ProductsOfInertia=[0 0 0]  ProductsOfInertiaUnits=kg*m^2  GraphicShininess=75  GraphicSpecularColor=[0.5 0.5 0.5 1.0]  GraphicVisPropType=SimpleVisualProperties
  Pin 1 : sm_lib/Body Elements/Cylindrical Solid  GraphicAmbientColor=[0.15 0.15 0.15 1.0]  BasedOnType=Density  CenterOfMass=[0 0 0]  CenterOfMassUnits=m  GraphicDiffuseColor=gray  CylinderLength=Dplates-Tplate  CylinderLengthUnits=m  CylinderRadius=RH1  CylinderRadiusUnits=m  Density=rhoSteel  DensityUnits=kg/(m^3)  DoExposeReferenceFrame=on  GraphicEmissiveColor=[0.0 0.0 0.0 1.0]  ExportEntireGeometry=off  SerializedFrames=<Frames/>  MarkerShape=Sphere  MarkerSize=10  GraphicType=FromGeometry  InertiaType=CalculateFromGeometry  Mass=1  MassUnits=kg  MomentsOfInertia=[1 1 1]  MomentsOfInertiaUnits=kg*m^2  GraphicOpacity=1.0  ProductsOfInertia=[0 0 0]  ProductsOfInertiaUnits=kg*m^2  GraphicShininess=75  GraphicSpecularColor=[0.5 0.5 0.5 1.0]  GraphicVisPropType=SimpleVisualProperties
  Pin 1 Transform : sm_lib/Frames and Transforms/Rigid Transform  TranslationMethod=Cartesian  TranslationStandardOffset=0  TranslationLengthUnit=m  TranslationStandardAxis=+Z  TranslationCartesianOffset=[L1 H1 Dplates/2]  TranslationROffset=0  TranslationROffsetUnits=m  TranslationZOffset=0  TranslationZOffsetUnits=m  TranslationThetaOffset=0  TranslationThetaOffsetUnits=deg  RotationMethod=None  RotationAngleUnits=deg  RotationStandardAxis=+Z  RotationAngle=0  RotationArbitraryAxis=[0 0 1]  FollAlignAxisA=+X  BaseAlignAxisA=+Y  FollAlignAxisB=+Y  BaseAlignAxisB=+Z  RotationSequenceAxes=FollowerAxes  RotationSequence=XYX  RotationSequenceAngles=[0 0 0]  RotationSequenceAnglesUnits=deg  RotationMatrix=[1 0 0; 0 1 0; 0 0 1]
  Pin 2 : sm_lib/Body Elements/Cylindrical Solid  GraphicAmbientColor=[0.15 0.15 0.15 1.0]  BasedOnType=Density  CenterOfMass=[0 0 0]  CenterOfMassUnits=m  GraphicDiffuseColor=gray  CylinderLength=Dplates-Tplate  CylinderLengthUnits=m  CylinderRadius=RH1  CylinderRadiusUnits=m  Density=rhoSteel  DensityUnits=kg/(m^3)  DoExposeReferenceFrame=on  GraphicEmissiveColor=[0.0 0.0 0.0 1.0]  ExportEntireGeometry=off  SerializedFrames=<Frames/>  MarkerShape=Sphere  MarkerSize=10  GraphicType=FromGeometry  InertiaType=CalculateFromGeometry  Mass=1  MassUnits=kg  MomentsOfInertia=[1 1 1]  MomentsOfInertiaUnits=kg*m^2  GraphicOpacity=1.0  ProductsOfInertia=[0 0 0]  ProductsOfInertiaUnits=kg*m^2  GraphicShininess=75  GraphicSpecularColor=[0.5 0.5 0.5 1.0]  GraphicVisPropType=SimpleVisualProperties
  Pin 2 Transform : sm_lib/Frames and Transforms/Rigid Transform  TranslationMethod=Cartesian  TranslationStandardOffset=0  TranslationLengthUnit=m  TranslationStandardAxis=+Z  TranslationCartesianOffset=[L2 H2 -Dplates/2]  TranslationROffset=0  TranslationROffsetUnits=m  TranslationZOffset=0  TranslationZOffsetUnits=m  TranslationThetaOffset=0  TranslationThetaOffsetUnits=deg  RotationMethod=None  RotationAngleUnits=deg  RotationStandardAxis=+Z  RotationAngle=0  RotationArbitraryAxis=[0 0 1]  FollAlignAxisA=+X  BaseAlignAxisA=+Y  FollAlignAxisB=+Y  BaseAlignAxisB=+Z  RotationSequenceAxes=FollowerAxes  RotationSequence=XYX  RotationSequenceAngles=[0 0 0]  RotationSequenceAnglesUnits=deg  RotationMatrix=[1 0 0; 0 1 0; 0 0 1]
  Plate-to-Bracket Transform : sm_lib/Frames and Transforms/Rigid Transform  TranslationMethod=Cartesian  TranslationStandardOffset=Dplates  TranslationLengthUnit=m  TranslationStandardAxis=-Z  TranslationCartesianOffset=[Dbracket Hbracket -Dplates/2]  TranslationROffset=0  TranslationROffsetUnits=m  TranslationZOffset=0  TranslationZOffsetUnits=m  TranslationThetaOffset=0  TranslationThetaOffsetUnits=deg  RotationMethod=AlignedAxes  RotationAngleUnits=deg  RotationStandardAxis=+Y  RotationAngle=90  RotationArbitraryAxis=[0 0 1]  FollAlignAxisA=+Y  BaseAlignAxisA=+Y  FollAlignAxisB=+Z  BaseAlignAxisB=+X  RotationSequenceAxes=FollowerAxes  RotationSequence=XYX  RotationSequenceAngles=[0 0 0]  RotationSequenceAnglesUnits=deg  RotationMatrix=[1 0 0; 0 1 0; 0 0 1]
  Plate-to-Plate Transform : sm_lib/Frames and Transforms/Rigid Transform  TranslationMethod=StandardAxis  TranslationStandardOffset=Dplates  TranslationLengthUnit=m  TranslationStandardAxis=-Z  TranslationCartesianOffset=[L1 H1 Tplate/2]  TranslationROffset=0  TranslationROffsetUnits=m  TranslationZOffset=0  TranslationZOffsetUnits=m  TranslationThetaOffset=0  TranslationThetaOffsetUnits=deg  RotationMethod=None  RotationAngleUnits=deg  RotationStandardAxis=+Z  RotationAngle=0  RotationArbitraryAxis=[0 0 1]  FollAlignAxisA=+X  BaseAlignAxisA=+Y  FollAlignAxisB=+Y  BaseAlignAxisB=+Z  RotationSequenceAxes=FollowerAxes  RotationSequence=XYX  RotationSequenceAngles=[0 0 0]  RotationSequenceAnglesUnits=deg  RotationMatrix=[1 0 0; 0 1 0; 0 0 1]
  Right Plate : sm_lib/Body Elements/Extruded Solid  GraphicAmbientColor=[0.15 0.15 0.15 1.0]  BasedOnType=Density  CenterOfMass=[0 0 0]  CenterOfMassUnits=m  GraphicDiffuseColor=hubColor  ExportConvexHullGeometry=off  ExtrusionCrossSection=plateSection  ExtrusionCrossSectionUnits=m  Density=rho  DensityUnits=kg/(m^3)  DoExposeReferenceFrame=on  GraphicEmissiveColor=[0.0 0.0 0.0 1.0]  ExportEntireGeometry=off  ExtrusionLength=Tplate  ExtrusionLengthUnits=m  ExtrusionType=General  SerializedFrames=<Frames/>  MarkerShape=Sphere  MarkerSize=10  GraphicType=FromGeometry  InertiaType=CalculateFromGeometry  Mass=1  MassUnits=kg  MomentsOfInertia=[1 1 1]  MomentsOfInertiaUnits=kg*m^2  PolygonNumSides=3  GraphicOpacity=1.0  PolygonOuterRadius=1  PolygonOuterRadiusUnits=m  ProductsOfInertia=[0 0 0]  ProductsOfInertiaUnits=kg*m^2  GraphicShininess=75  GraphicSpecularColor=[0.5 0.5 0.5 1.0]  GraphicVisPropType=SimpleVisualProperties
  Lower Arm : PMIOPort  Side=Left
  Cylinder Base [Lower Joint] : PMIOPort  Port=2  Side=Left
  Bracket : PMIOPort  Port=3  Side=Right
  Attachment Arm Left : PMIOPort  Port=4  Side=Left
  Attachment Arm Right : PMIOPort  Port=5  Side=Right
  connections:
  Cylinder Transform/RConn1 -- Cylinder Base [Lower Joint]/RConn1
  Attachment Arm Right/RConn1 -- Attachment Arm Transform Right/RConn1
  Attachment Arm Left/RConn1 -- Attachment Arm Transform Left/RConn1
  Pin 2 Transform/RConn1 -- Cylinder Transform/LConn1 -- Pin 2/RConn1
  Bracket/RConn1 -- Plate-to-Bracket Transform/RConn1
  Lower Arm/RConn1 -- Pin 1/RConn1 -- Pin 1 Transform/RConn1
  Plate-to-Plate Transform/LConn1 -- Pin 2 Transform/LConn1 -- Plate-to-Bracket Transform/LConn1 -- Attachment Arm Transform Left/LConn1 -- Left Plate/RConn1
  Plate-to-Plate Transform/RConn1 -- Right Plate/RConn1 -- Attachment Arm Transform Right/LConn1 -- Pin 1 Transform/LConn1
